simulink model "RMXENCODER"  (R2026a)
settings: Solver=FixedStepAuto  StopTime=inf  FixedStep=0.001
undefined symbols (not defined in the file): Blocking, Non
libraries: amg_usbconverter_n_connect_lib x2
settings Model: Creator=pboon  LastModifiedBy=samli

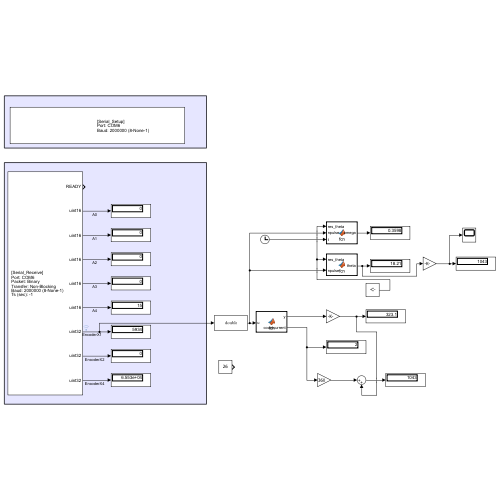
[thumbnail: Simulink's stored preview of the top-level diagram]
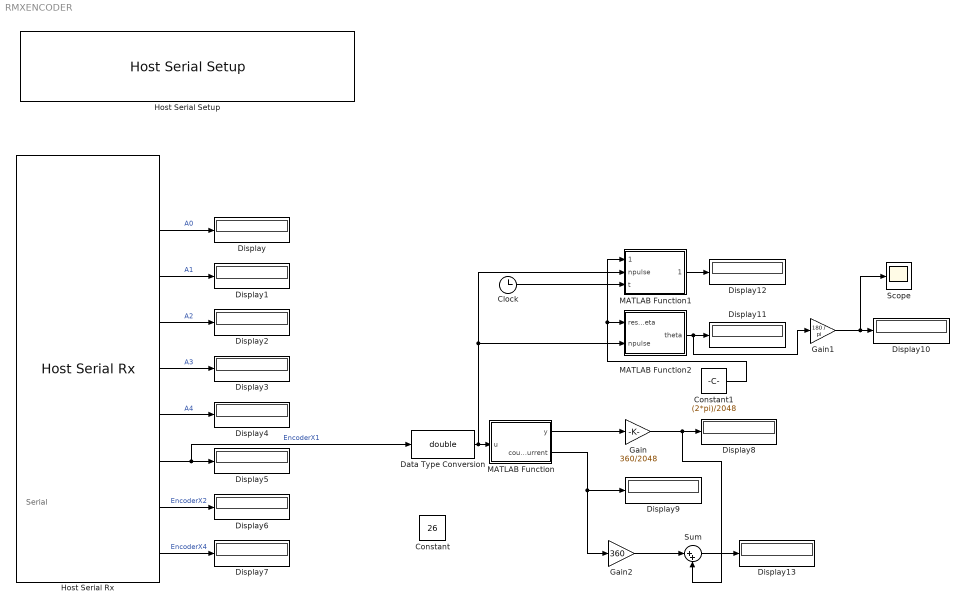
== system RMXENCODER ==
  note: Serial
  Clock : Clock
  Constant : Constant  Value=26
  Constant1 : Constant  Value=(2*pi)/2048
  Data Type Conversion : DataTypeConversion  OutDataTypeStr=double  SaturateOnIntegerOverflow=off  RndMeth=Floor
  Display{,1..13} (14 alike) : Display
  Gain : Gain  Gain=360/2048
  Gain1 : Gain  Gain=180 / pi
  Gain2 : Gain  Gain=360
  Host Serial Rx : amg_usbconverter_n_connect_lib/Host Serial Rx  conf=rx  port=COM6  baudrate=2000000  databits=8  parity=None  stopbit=1  flowcontrol=None  transfer=Non-Blocking  timeout=5  packetmode=Binary  enableinitialvalues=off  initialvalues=[]  binheader='25'  binterminator='4E 4E'  porttype_double=0  porttype_single=0  porttype_int8=0  porttype_uint8=0  porttype_int16=0  porttype_uint16=5  porttype_int32=0  porttype_uint32=3  asciiformat='%d,%f'  rx_asciiterminator="CRLF (0x0D 0x0A - \"\\r\\n\")"  tx_asciiterminator="CRLF (0x0D 0x0A - \"\\r\\n\")"  sampletime=0.001  enablecustomportlabel=off  cinputportlabel=0  coutputportlabel=A  portpinstr=0  blockid=HostSerialRx  inputporttype=[]  inputportwidth=[]  inputportlabel={}  outputporttype=[3 5 5 5 5 5 7 7 7]  outputportwidth=[1 1 1 1 1 1 1 1 1]  outputportlabel={'READY','uint16','uint16','uint16','uint16','uint16','uint32','uint32','uint32'}  compat=0  optionstring=[]  autoport='COM6'
  Host Serial Setup : amg_usbconverter_n_connect_lib/Host Serial Setup  conf=setup  port=COM6  baudrate=2000000  databits=8  parity=None  stopbit=1  flowcontrol=None  transfer=Blocking  timeout=2  packetmode=Binary  initialvalues=[]  binheader='7E 7E'  binterminator='03 03'  porttype_double=0  porttype_single=1  porttype_int8=0  porttype_uint8=0  porttype_int16=0  porttype_uint16=0  porttype_int32=0  porttype_uint32=2  asciiformat='%d %u %x'  rx_asciiterminator="CRLF (0x0D 0x0A - \"\\r\\n\")"  tx_asciiterminator="CRLF (0x0D 0x0A - \"\\r\\n\")"  sampletime=-1  enablecustomportlabel=off  cinputportlabel=0  coutputportlabel=A  portpinstr=0  blockid=HostSerialSetup  inputporttype=[]  inputportwidth=[]  inputportlabel={}  outputporttype=[]  outputportwidth=[]  outputportlabel={}  compat=0  optionstring=[]  autoport='COM6'
  MATLAB Function : MATLAB Function  TreatAsAtomicUnit=on
  MATLAB Function1 : MATLAB Function  TreatAsAtomicUnit=on
  MATLAB Function2 : MATLAB Function  TreatAsAtomicUnit=on
  Scope : Scope
      settings: ActiveDisplayYMinimum=-610.71095916778427  ActiveDisplayYMaximum=999.345844846393
  Sum : Sum  Inputs=|++
  wires:
  Host Serial Rx/2 -> Display/1  "A0"
  Host Serial Rx/3 -> Display1/1  "A1"
  Host Serial Rx/4 -> Display2/1  "A2"
  Host Serial Rx/5 -> Display3/1  "A3"
  Host Serial Rx/6 -> Display4/1  "A4"
  Host Serial Rx/7 -> Data Type Conversion/1, Display5/1  "EncoderX1"
  Host Serial Rx/8 -> Display6/1  "EncoderX2"
  Host Serial Rx/9 -> Display7/1  "EncoderX4"
  MATLAB Function/2(countcurrent) -> Gain2/1, Display9/1
  MATLAB Function/1(y) -> Gain/1
  Gain/1 -> Sum/2, Display8/1
  MATLAB Function2/1(theta) -> Gain1/1, Display11/1
  Constant1/1 -> MATLAB Function1/1(res_theta), MATLAB Function2/1(res_theta)
  Gain1/1 -> Scope/1, Display10/1
  Clock/1 -> MATLAB Function1/3(t)
  MATLAB Function1/1(omega) -> Display12/1
  Data Type Conversion/1 -> MATLAB Function1/2(npulse), MATLAB Function2/2(npulse), MATLAB Function/1(u)
  Gain2/1 -> Sum/1
  Sum/1 -> Display13/1

== matlab function RMXENCODER/MATLAB Function1 ==
  data: res_theta input; omega output; npulse input; t input
function omega = fcn(res_theta, npulse, t)

if t <= 0
    omega = 0;
else
    theta = res_theta * npulse;
    omega = theta / t;
end

end

== matlab function RMXENCODER/MATLAB Function ==
  data: u input; y output; countcurrent output
function [y, countcurrent] = fcn(u)

countcurrent = floor(u / 2048);

y = mod(u, 2048);

end

== matlab function RMXENCODER/MATLAB Function2 ==
  data: res_theta input; theta output; npulse input
function theta = fcn(res_theta, npulse)

theta = res_theta * npulse;

end
